simulink model "togi_pll"  (R2023b)
settings: Solver=VariableStepAuto  StartTime=0.0  StopTime=10.0  RelTol=1e-3
libraries: spsAlphaBetaZerotodq0Lib x1
settings Model: Creator=sabar  LastModifiedBy=sabar

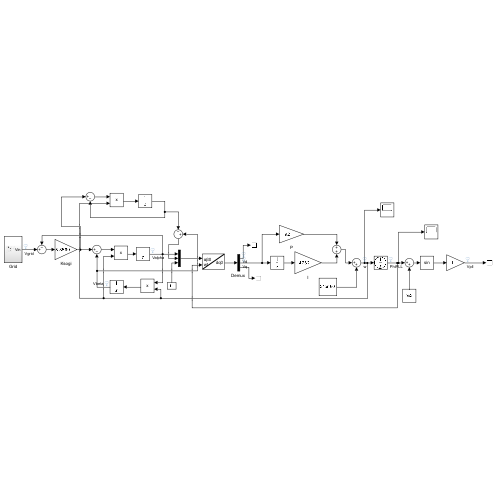
[thumbnail: Simulink's stored preview of the top-level diagram]
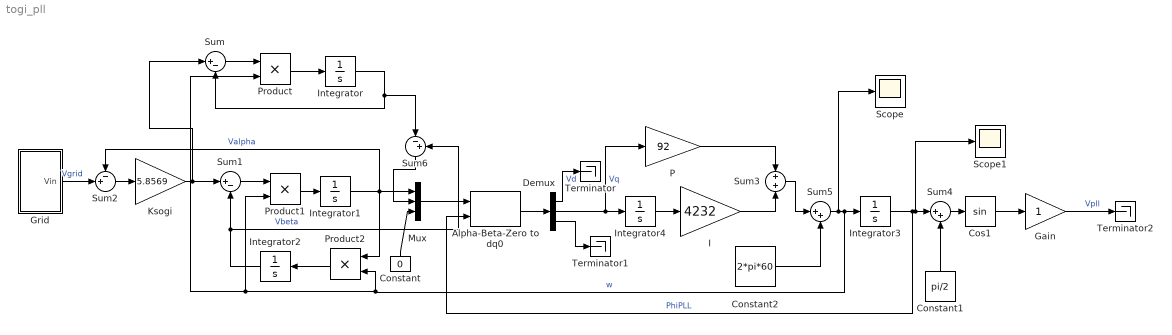
== system togi_pll ==
  Alpha-Beta-Zero to dq0 : spsAlphaBetaZerotodq0Lib/Alpha-Beta-Zero to dq0  Alignment=Aligned with phase A axis
  Constant : Constant  Value=0
  Constant1 : Constant  Value=pi/2
  Constant2 : Constant  Value=2*pi*60
  Cos1 : Trigonometry
  "Demux " : Demux  Outputs=3
  Gain : Gain
  Grid : Subsystem
  I : Gain  Gain=4232
  Integrator : Integrator
  Integrator1 : Integrator  UpperSaturationLimit=1e3  LowerSaturationLimit=-1e3
  Integrator2 : Integrator  UpperSaturationLimit=1e3  LowerSaturationLimit=-1e3
  Integrator3 : Integrator  WrapState=on
  Integrator4 : Integrator
  Ksogi : Gain  Gain=5.8569
  Mux : Mux  Inputs=3
  P : Gain  Gain=92
  Product : Product
  Product1 : Product
  Product2 : Product
  Scope : Scope
  Scope1 : Scope
  Sum : Sum  Inputs=|+-
  Sum1 : Sum  Inputs=|+-
  Sum2 : Sum  Inputs=-+|
  Sum3 : Sum  Inputs=+|+
  Sum4 : Sum  Inputs=|++
  Sum5 : Sum  Inputs=|++
  Sum6 : Sum  Inputs=|-+
  Terminator : Terminator
  Terminator1 : Terminator
  Terminator2 : Terminator
  wires:
  Sum/1 -> Product/1
  Grid/1(Vin) -> Sum2/2  "Vgrid"
  Ksogi/1 -> Sum/1, Sum1/1
  P/1 -> Sum3/1
  Constant1/1 -> Sum4/2
  "Demux "/1 -> Terminator/1  "Vd"
  Gain/1 -> Terminator2/1  "Vpll"
  I/1 -> Sum3/2
  Sum2/1 -> Ksogi/1
  Integrator1/1 -> Product2/1, Mux/1, Sum2/1  "Valpha"
  Mux/1 -> Alpha-Beta-Zero to dq0/1
  Sum1/1 -> Product1/1
  Integrator2/1 -> Sum6/2, Sum1/2  "Vbeta"
  "Demux "/3 -> Terminator1/1
  Alpha-Beta-Zero to dq0/1 -> "Demux "/1
  Integrator3/1 -> Scope1/1, Sum4/1, Alpha-Beta-Zero to dq0/2  "PhiPLL"
  Product2/1 -> Integrator2/1
  Integrator4/1 -> I/1
  Constant2/1 -> Sum5/2
  Sum4/1 -> Cos1/1
  "Demux "/2 -> P/1, Integrator4/1  "Vq"
  Sum5/1 -> Scope/1, Product/2, Product1/2, Product2/2, Integrator3/1  "w"
  Product1/1 -> Integrator1/1
  Cos1/1 -> Gain/1
  Constant/1 -> Mux/3
  Sum3/1 -> Sum5/1
  Product/1 -> Integrator/1
  Integrator/1 -> Sum6/1, Sum/2
  Sum6/1 -> Mux/2

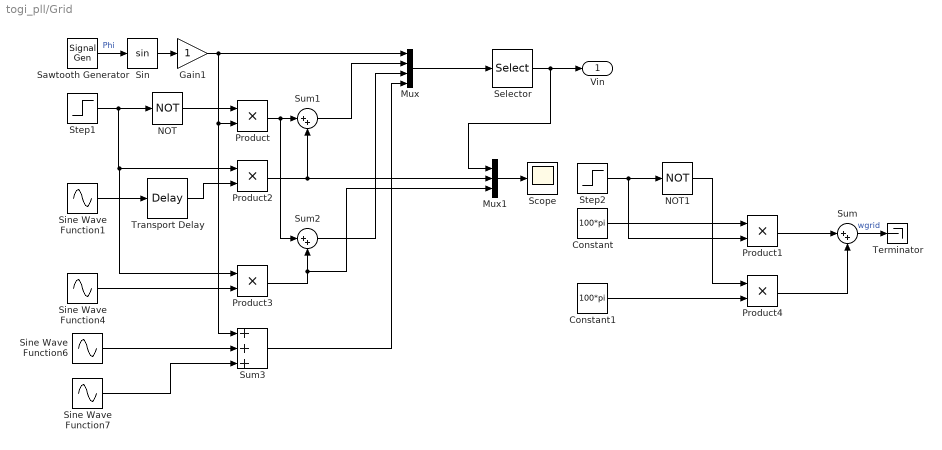
== system togi_pll/Grid ==
  Constant : Constant  Value=100*pi
  Constant1 : Constant  Value=100*pi
  Gain1 : Gain
  Mux : Mux
  Mux1 : Mux  Inputs=3
  NOT : Logic  Operator=NOT  IconShape=distinctive  AllPortsSameDT=off  OutDataTypeStr=boolean
  NOT1 : Logic  Operator=NOT  IconShape=distinctive  AllPortsSameDT=off  OutDataTypeStr=boolean
  Product{,1..4} (5 alike) : Product
  Sawtooth Generator : SignalGenerator  WaveForm=sawtooth  Amplitude=pi  Frequency=314.159  Units=rad/sec
  Scope : Scope
  Selector : Selector  InputPortWidth=4  IndexOptions=Index vector (dialog)  Indices=1  OutputSizes=1
  Sin : Trigonometry
  Sine Wave Function1 : Sin  Frequency=314.159  SampleTime=0
  Sine Wave Function4 : Sin  Frequency=314.159  Phase=pi  SampleTime=0
  Sine Wave Function6 : Sin  Amplitude=1*0.1  Frequency=5*100*pi  SampleTime=0
  Sine Wave Function7 : Sin  Amplitude=1*0.05  Frequency=10*100*pi  SampleTime=0
  Step1 : Step  SampleTime=0
  Step2 : Step  Before=1  After=0  SampleTime=0
  Sum : Sum  Inputs=|++
  Sum1 : Sum  Inputs=|++
  Sum2 : Sum  Inputs=|++
  Sum3 : Sum  Inputs=+++
  Terminator : Terminator
  Transport Delay : TransportDelay  DelayTime=1000e-3
  Vin : Outport
  wires:
  Transport Delay/1 -> Product2/2
  Sine Wave Function7/1 -> Sum3/3
  Sum/1 -> Terminator/1  "wgrid"
  Sum3/1 -> Mux/4
  Constant/1 -> Product1/1
  Sine Wave Function1/1 -> Transport Delay/1
  Sin/1 -> Gain1/1
  Sum2/1 -> Mux/3
  Sawtooth Generator/1 -> Sin/1  "Phi"
  Product3/1 -> Mux1/3, Sum2/2
  Step2/1 -> Product1/2, NOT1/1
  Sine Wave Function4/1 -> Product3/2
  NOT1/1 -> Product4/1
  Sine Wave Function6/1 -> Sum3/2
  Mux/1 -> Selector/1
  Mux1/1 -> Scope/1
  NOT/1 -> Product/1
  Gain1/1 -> Sum3/1, Product/2, Mux/1
  Product2/1 -> Mux1/2, Sum1/2
  Product/1 -> Sum2/1, Sum1/1
  Step1/1 -> Product3/1, Product2/1, NOT/1
  Product1/1 -> Sum/1
  Sum1/1 -> Mux/2
  Selector/1 -> Mux1/1, Vin/1
  Product4/1 -> Sum/2
  Constant1/1 -> Product4/2
